simulink model "pendulum_2d_control_simulation"  (R2017a)
settings: Solver=FixedStepAuto  StartTime=0.0  StopTime=15  FixedStep=dt  RelTol=1e-3
values from neighbouring files (symbols this model uses):
  A = [0, 1, 0, 0 ... (first row only)    [formPendel.m]    (also in initialize_controller_pendulum2d.m = double(subs(A_sym)))
  B = [0, 1, 0, -1/L]'    [formPendel.m]    (also in initialize_controller_pendulum2d.m = double(subs(B_sym)))
  C = [1, 0, 0, 0 ... (first row only)    [formPendel.m]    (also in initialize_controller_pendulum2d.m = double(subs(C_sym)))
  D = [0,0]'    [formPendel.m]    (also in initialize_controller_pendulum2d.m = double(subs(D_sym)))
  dt = 1e-3    (= 0.001)    [fJacobian_simulink.m]    (also in formPendel.m; initialize_controller_pendulum2d.m)
  K = lqr(A,B,Q_lqr, R_lqr)    [formPendel.m]    (also in initialize_controller_pendulum2d.m = lqr(A,B,Q_LQR, R_LQR))
  Ke = -KI(1)    [initialize_controller_pendulum2d.m]
  Ko = KI(2:5)    [initialize_controller_pendulum2d.m]
  N = inv(Cm*inv(B*K - A)*B)    [initialize_controller_pendulum2d.m]
  R = diag([0.001^2, 0.01^2])    [formPendel.m]    (also in initialize_controller_pendulum2d.m)
  theta_init = 10*pi/180    (= 0.174532925199)    [formPendel.m]    (also in initialize_controller_pendulum2d.m = 0.349065850399)
  x0 = [0; 0; 0; 0]    [initialize_controller_pendulum2d.m]
  x_init = 0    [formPendel.m]    (also in initialize_controller_pendulum2d.m)
undefined symbols (not defined in the file or in its folder): Continuous, Time
libraries: sharedTrackingLibrary x3, ctrlSharedLib x1
settings Model: Creator=Workstation  LastModifiedBy=Jan

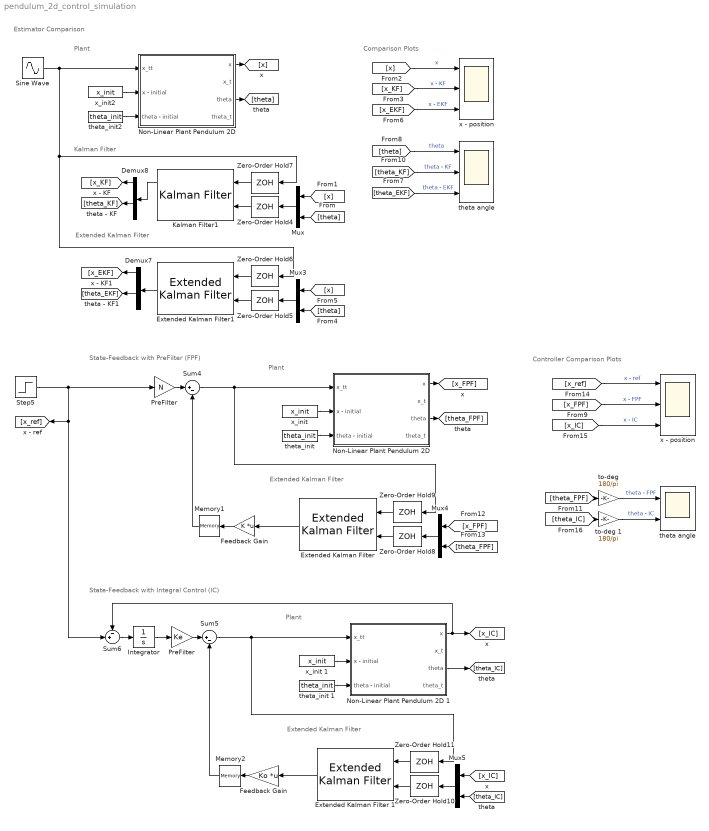
== system pendulum_2d_control_simulation ==
  note: Controller Comparison Plots
  note: Estimator Comparison
  note: State-Feedback with PreFilter (FPF)
  note: Comparison Plots
  note: Extended Kalman Filter
  note: Kalman Filter
  note: Plant
  note: Extended Kalman Filter
  note: Plant
  note: State-Feedback with Integral Control (IC)
  note: Extended Kalman Filter
  note: Plant
  " PreFilter " : Gain  Gain=Ke
  Demux7 : Demux
  Demux8 : Demux
  "Extended Kalman Filter " : sharedTrackingLibrary/Extended Kalman Filter  StateTransitionFcn=f_simulink  HasStateTransitionJacobianFcn=off  HasAdditiveProcessNoise=Additive  ProcessNoise=Q  HasTimeVaryingProcessNoise=off  HasStateTransitionFcnExtraArgument=1  InitialState=x0  InitialStateCovariance=P  MeasurementFcn1=h_simulink  HasMeasurementJacobianFcn1=off  HasMeasurementEnablePort1=off  HasAdditiveMeasurementNoise1=Additive  MeasurementNoise1=R  HasTimeVaryingMeasurementNoise1=off  HasMeasurementFcnExtraArgument1=0  MeasurementFcn2=myMeasurementFcn  HasMeasurementJacobianFcn2=off  HasMeasurementEnablePort2=off  HasAdditiveMeasurementNoise2=Additive  MeasurementNoise2=1  HasTimeVaryingMeasurementNoise2=off  HasMeasurementFcnExtraArgument2=0  MeasurementFcn3=myMeasurementFcn  HasMeasurementJacobianFcn3=off  HasMeasurementEnablePort3=off  HasAdditiveMeasurementNoise3=Additive  MeasurementNoise3=1  HasTimeVaryingMeasurementNoise3=off  HasMeasurementFcnExtraArgument3=0  MeasurementFcn4=myMeasurementFcn  HasMeasurementJacobianFcn4=off  HasMeasurementEnablePort4=off  HasAdditiveMeasurementNoise4=Additive  MeasurementNoise4=1  HasTimeVaryingMeasurementNoise4=off  HasMeasurementFcnExtraArgument4=0  MeasurementFcn5=myMeasurementFcn  HasMeasurementJacobianFcn5=off  HasMeasurementEnablePort5=off  HasAdditiveMeasurementNoise5=Additive  MeasurementNoise5=1  HasTimeVaryingMeasurementNoise5=off  HasMeasurementFcnExtraArgument5=0  EnableMultirate=off  StateTransitionFcnSampleTime=1  MeasurementFcn1SampleTime=1  MeasurementFcn2SampleTime=1  MeasurementFcn3SampleTime=1  MeasurementFcn4SampleTime=1  MeasurementFcn5SampleTime=1  UseCurrentEstimator=on  OutputStateCovariance=off  DataType=double  SampleTime=dt  NumberOfMeasurements=1
  Extended Kalman Filter 1 : sharedTrackingLibrary/Extended Kalman Filter  StateTransitionFcn=f_simulink  HasStateTransitionJacobianFcn=off  HasAdditiveProcessNoise=Additive  ProcessNoise=Q  HasTimeVaryingProcessNoise=off  HasStateTransitionFcnExtraArgument=1  InitialState=x0  InitialStateCovariance=P  MeasurementFcn1=h_simulink  HasMeasurementJacobianFcn1=off  HasMeasurementEnablePort1=off  HasAdditiveMeasurementNoise1=Additive  MeasurementNoise1=R  HasTimeVaryingMeasurementNoise1=off  HasMeasurementFcnExtraArgument1=0  MeasurementFcn2=myMeasurementFcn  HasMeasurementJacobianFcn2=off  HasMeasurementEnablePort2=off  HasAdditiveMeasurementNoise2=Additive  MeasurementNoise2=1  HasTimeVaryingMeasurementNoise2=off  HasMeasurementFcnExtraArgument2=0  MeasurementFcn3=myMeasurementFcn  HasMeasurementJacobianFcn3=off  HasMeasurementEnablePort3=off  HasAdditiveMeasurementNoise3=Additive  MeasurementNoise3=1  HasTimeVaryingMeasurementNoise3=off  HasMeasurementFcnExtraArgument3=0  MeasurementFcn4=myMeasurementFcn  HasMeasurementJacobianFcn4=off  HasMeasurementEnablePort4=off  HasAdditiveMeasurementNoise4=Additive  MeasurementNoise4=1  HasTimeVaryingMeasurementNoise4=off  HasMeasurementFcnExtraArgument4=0  MeasurementFcn5=myMeasurementFcn  HasMeasurementJacobianFcn5=off  HasMeasurementEnablePort5=off  HasAdditiveMeasurementNoise5=Additive  MeasurementNoise5=1  HasTimeVaryingMeasurementNoise5=off  HasMeasurementFcnExtraArgument5=0  EnableMultirate=off  StateTransitionFcnSampleTime=1  MeasurementFcn1SampleTime=1  MeasurementFcn2SampleTime=1  MeasurementFcn3SampleTime=1  MeasurementFcn4SampleTime=1  MeasurementFcn5SampleTime=1  UseCurrentEstimator=on  OutputStateCovariance=off  DataType=double  SampleTime=dt  NumberOfMeasurements=1
  Extended Kalman Filter1 : sharedTrackingLibrary/Extended Kalman Filter  StateTransitionFcn=f_simulink  HasStateTransitionJacobianFcn=off  HasAdditiveProcessNoise=Additive  ProcessNoise=Q  HasTimeVaryingProcessNoise=off  HasStateTransitionFcnExtraArgument=1  InitialState=x0  InitialStateCovariance=P  MeasurementFcn1=h_simulink  HasMeasurementJacobianFcn1=off  HasMeasurementEnablePort1=off  HasAdditiveMeasurementNoise1=Additive  MeasurementNoise1=R  HasTimeVaryingMeasurementNoise1=off  HasMeasurementFcnExtraArgument1=0  MeasurementFcn2=myMeasurementFcn  HasMeasurementJacobianFcn2=off  HasMeasurementEnablePort2=off  HasAdditiveMeasurementNoise2=Additive  MeasurementNoise2=1  HasTimeVaryingMeasurementNoise2=off  HasMeasurementFcnExtraArgument2=0  MeasurementFcn3=myMeasurementFcn  HasMeasurementJacobianFcn3=off  HasMeasurementEnablePort3=off  HasAdditiveMeasurementNoise3=Additive  MeasurementNoise3=1  HasTimeVaryingMeasurementNoise3=off  HasMeasurementFcnExtraArgument3=0  MeasurementFcn4=myMeasurementFcn  HasMeasurementJacobianFcn4=off  HasMeasurementEnablePort4=off  HasAdditiveMeasurementNoise4=Additive  MeasurementNoise4=1  HasTimeVaryingMeasurementNoise4=off  HasMeasurementFcnExtraArgument4=0  MeasurementFcn5=myMeasurementFcn  HasMeasurementJacobianFcn5=off  HasMeasurementEnablePort5=off  HasAdditiveMeasurementNoise5=Additive  MeasurementNoise5=1  HasTimeVaryingMeasurementNoise5=off  HasMeasurementFcnExtraArgument5=0  EnableMultirate=off  StateTransitionFcnSampleTime=1  MeasurementFcn1SampleTime=1  MeasurementFcn2SampleTime=1  MeasurementFcn3SampleTime=1  MeasurementFcn4SampleTime=1  MeasurementFcn5SampleTime=1  UseCurrentEstimator=on  OutputStateCovariance=off  DataType=double  SampleTime=dt  NumberOfMeasurements=1
  Feedback Gain : Gain  Gain=Ko  Multiplication=Matrix(K*u)
  "Feedback Gain " : Gain  Gain=K  Multiplication=Matrix(K*u)
  Integrator : Integrator
  Kalman Filter1 : ctrlSharedLib/Kalman Filter  TimeDomain=Continuous-Time  UseCurrentEstimator=off  ModelSource=Individual A, B, C, D matrices  ModelSourceVariable=ss(0.95,1,1,0,1)  A=A  B=B  C=C  D=D  NumberOfStates=1  NumberOfInputs=1  NumberOfOutputs=1  InitialEstimateSource=Dialog  X0=x0  P0=10  UseK=off  UseGH=off  NumberOfProcessNoiseInputs=1  G=1  TimeInvariantG=on  H=0  TimeInvariantH=on  Q=Q  TimeInvariantQ=on  R=R  TimeInvariantR=on  N=0  TimeInvariantN=on  AddInputPort=on  AddEnablePort=off  ExternalReset=none  OutputEstimatedY=on  OutputP=off  Ts=dt
  Memory1 : Memory
  Memory2 : Memory
  Mux{,3..5} (4 alike) : Mux  Inputs=2
  Non-Linear Plant Pendulum 2D : Subsystem
  "Non-Linear Plant Pendulum 2D " : Subsystem
  Non-Linear Plant Pendulum 2D 1 : Subsystem
  PreFilter : Gain  Gain=N
  Sine Wave : Sin  SampleTime=0
  Step5 : Step  Time=0  SampleTime=0
  Sum4 : Sum  Inputs=|+-
  Sum5 : Sum  Inputs=|+-
  Sum6 : Sum  Inputs=-+|
  Zero-Order Hold{5..6,8..11} (6 alike) : ZeroOrderHold  SampleTime=dt
  Zero-Order Hold4 : ZeroOrderHold  SampleTime=-1
  Zero-Order Hold7 : ZeroOrderHold  SampleTime=-1
  theta angle : Scope  NumInputPorts=3
  "theta angle " : Scope  NumInputPorts=2
  "theta_init " : Constant  Value=theta_init
  theta_init 1 : Constant  Value=theta_init
  theta_init2 : Constant  Value=theta_init
  "to-deg " : Gain  Gain=180/pi
  to-deg 1 : Gain  Gain=180/pi
  x - position : Scope  NumInputPorts=3
  "x - position " : Scope  NumInputPorts=3
  "x_init " : Constant  Value=x_init
  x_init 1 : Constant  Value=x_init
  x_init2 : Constant  Value=x_init
  wires:
  x_init2/1 -> Non-Linear Plant Pendulum 2D/2(x - initial)
  theta_init2/1 -> Non-Linear Plant Pendulum 2D/3(theta - initial)
  Non-Linear Plant Pendulum 2D/3(theta) -> [theta]
  Non-Linear Plant Pendulum 2D/1(x) -> [x]
  Mux/1 -> Zero-Order Hold4/1
  Zero-Order Hold4/1 -> Kalman Filter1/2
  [theta] -> Mux/2
  [x] -> Mux/1
  [x] -> x - position/1  "x"
  [x_KF] -> x - position/2  "x - KF"
  Zero-Order Hold5/1 -> Extended Kalman Filter1/2
  [x] -> Mux3/1
  [theta] -> Mux3/2
  Mux3/1 -> Zero-Order Hold5/1
  Extended Kalman Filter1/1 -> Demux7/1
  Demux7/1 -> [x_EKF]
  [x_EKF] -> x - position/3  "x - EKF"
  Demux7/3 -> [theta_EKF]
  Kalman Filter1/1 -> Demux8/1
  Demux8/1 -> [x_KF]
  Demux8/3 -> [theta_KF]
  Zero-Order Hold7/1 -> Kalman Filter1/1
  Zero-Order Hold6/1 -> Extended Kalman Filter1/1
  Sine Wave/1 -> Non-Linear Plant Pendulum 2D/1(x_tt), Zero-Order Hold6/1, Zero-Order Hold7/1
  [theta_KF] -> theta angle/2  "theta - KF"
  [theta_EKF] -> theta angle/3  "theta - EKF"
  [theta] -> theta angle/1  "theta"
  Zero-Order Hold9/1 -> "Extended Kalman Filter "/1
  "Extended Kalman Filter "/1 -> "Feedback Gain "/1
  Mux4/1 -> Zero-Order Hold8/1
  [theta_FPF] -> Mux4/2
  [x_FPF] -> Mux4/1
  Zero-Order Hold8/1 -> "Extended Kalman Filter "/2
  "Non-Linear Plant Pendulum 2D "/1(x) -> [x_FPF]
  "Non-Linear Plant Pendulum 2D "/3(theta) -> [theta_FPF]
  "theta_init "/1 -> "Non-Linear Plant Pendulum 2D "/3(theta - initial)
  "x_init "/1 -> "Non-Linear Plant Pendulum 2D "/2(x - initial)
  Sum4/1 -> Zero-Order Hold9/1, "Non-Linear Plant Pendulum 2D "/1(x_tt)
  "Feedback Gain "/1 -> Memory1/1
  Memory1/1 -> Sum4/2
  PreFilter/1 -> Sum4/1
  [theta_FPF] -> "to-deg "/1
  [x_FPF] -> "x - position "/2  "x - FPF"
  [x_ref] -> "x - position "/1  "x - ref"
  "to-deg "/1 -> "theta angle "/1  "theta - FPF"
  Integrator/1 -> " PreFilter "/1
  " PreFilter "/1 -> Sum5/1
  Memory2/1 -> Sum5/2
  Feedback Gain/1 -> Memory2/1
  Sum5/1 -> Non-Linear Plant Pendulum 2D 1/1(x_tt), Zero-Order Hold11/1
  x_init 1/1 -> Non-Linear Plant Pendulum 2D 1/2(x - initial)
  theta_init 1/1 -> Non-Linear Plant Pendulum 2D 1/3(theta - initial)
  Non-Linear Plant Pendulum 2D 1/3(theta) -> [theta_IC]
  Zero-Order Hold10/1 -> Extended Kalman Filter 1/2
  [x_IC] -> Mux5/1
  [theta_IC] -> Mux5/2
  Mux5/1 -> Zero-Order Hold10/1
  Extended Kalman Filter 1/1 -> Feedback Gain/1
  Zero-Order Hold11/1 -> Extended Kalman Filter 1/1
  Sum6/1 -> Integrator/1
  Non-Linear Plant Pendulum 2D 1/1(x) -> [x_IC], Sum6/1
  [x_IC] -> "x - position "/3  "x - IC"
  [theta_IC] -> to-deg 1/1
  to-deg 1/1 -> "theta angle "/2  "theta - IC"
  Step5/1 -> PreFilter/1, [x_ref], Sum6/2

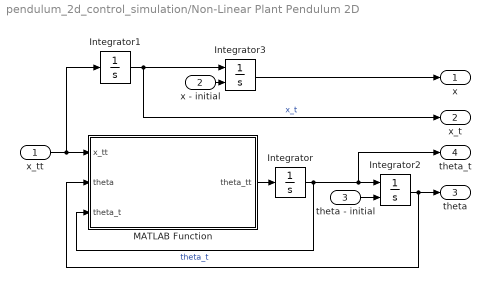
== system pendulum_2d_control_simulation/Non-Linear Plant Pendulum 2D ==
  x_tt : Inport
  x - initial : Inport  Port=2
  theta - initial : Inport  Port=3
  Integrator : Integrator
  Integrator1 : Integrator
  Integrator2 : Integrator  InitialConditionSource=external
  Integrator3 : Integrator  InitialConditionSource=external
  MATLAB Function : MATLAB Function  TreatAsAtomicUnit=on
  x : Outport
  x_t : Outport  Port=2
  theta : Outport  Port=3
  theta_t : Outport  Port=4
  wires:
  Integrator/1 -> MATLAB Function/3(theta_t), theta_t/1, Integrator2/1  "theta_t"
  x_tt/1 -> MATLAB Function/1(x_tt), Integrator1/1
  x - initial/1 -> Integrator3/2
  Integrator1/1 -> Integrator3/1, x_t/1  "x_t"
  MATLAB Function/1(theta_tt) -> Integrator/1
  theta - initial/1 -> Integrator2/2
  Integrator2/1 -> MATLAB Function/2(theta), theta/1
  Integrator3/1 -> x/1

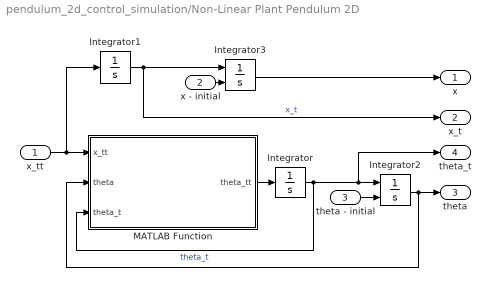
== system pendulum_2d_control_simulation/Non-Linear Plant Pendulum 2D  ==
  x_tt : Inport
  x - initial : Inport  Port=2
  theta - initial : Inport  Port=3
  Integrator : Integrator
  Integrator1 : Integrator
  Integrator2 : Integrator  InitialConditionSource=external
  Integrator3 : Integrator  InitialConditionSource=external
  MATLAB Function : MATLAB Function  TreatAsAtomicUnit=on
  x : Outport
  x_t : Outport  Port=2
  theta : Outport  Port=3
  theta_t : Outport  Port=4
  wires:
  Integrator3/1 -> x/1
  Integrator2/1 -> theta/1, MATLAB Function/2(theta)
  theta - initial/1 -> Integrator2/2
  MATLAB Function/1(theta_tt) -> Integrator/1
  Integrator1/1 -> x_t/1, Integrator3/1  "x_t"
  x - initial/1 -> Integrator3/2
  x_tt/1 -> Integrator1/1, MATLAB Function/1(x_tt)
  Integrator/1 -> Integrator2/1, theta_t/1, MATLAB Function/3(theta_t)  "theta_t"

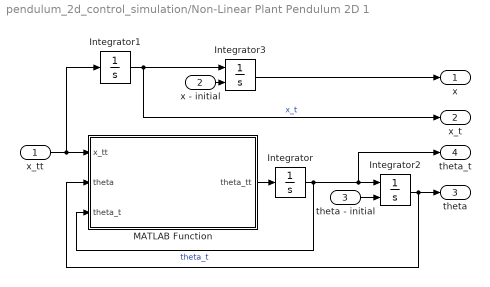
== system pendulum_2d_control_simulation/Non-Linear Plant Pendulum 2D 1 ==
  x_tt : Inport
  x - initial : Inport  Port=2
  theta - initial : Inport  Port=3
  Integrator : Integrator
  Integrator1 : Integrator
  Integrator2 : Integrator  InitialConditionSource=external
  Integrator3 : Integrator  InitialConditionSource=external
  MATLAB Function : MATLAB Function  TreatAsAtomicUnit=on
  x : Outport
  x_t : Outport  Port=2
  theta : Outport  Port=3
  theta_t : Outport  Port=4
  wires:
  Integrator/1 -> MATLAB Function/3(theta_t), theta_t/1, Integrator2/1  "theta_t"
  x_tt/1 -> MATLAB Function/1(x_tt), Integrator1/1
  x - initial/1 -> Integrator3/2
  Integrator1/1 -> Integrator3/1, x_t/1  "x_t"
  MATLAB Function/1(theta_tt) -> Integrator/1
  theta - initial/1 -> Integrator2/2
  Integrator2/1 -> MATLAB Function/2(theta), theta/1
  Integrator3/1 -> x/1

== matlab function pendulum_2d_control_simulation/Non-Linear Plant Pendulum 2D/MATLAB Function ==
  data: x_tt input; theta input; theta_tt output; theta_t input
function theta_tt = pendulum_dynamics(x_tt, theta, theta_t)
    
    % Constants
    g = 9.81;   % Gravity
    L = 2.0;    % Wire length
    
    % Pendulum ODE
    theta_tt = (-g*sin(theta) - cos(theta)*x_tt)/(L);

== matlab function pendulum_2d_control_simulation/Non-Linear Plant Pendulum 2D /MATLAB Function ==
  data: x_tt input; theta input; theta_tt output; theta_t input
function theta_tt = pendulum_dynamics(x_tt, theta, theta_t)
    
    % Constants
    g = 9.81;   % Gravity
    L = 2.0;    % Wire length
    
    % Pendulum ODE
    theta_tt = (-g*sin(theta) - cos(theta)*x_tt)/(L);

== matlab function pendulum_2d_control_simulation/Non-Linear Plant Pendulum 2D 1/MATLAB Function ==
  data: x_tt input; theta input; theta_tt output; theta_t input
function theta_tt = pendulum_dynamics(x_tt, theta, theta_t)
    
    % Constants
    g = 9.81;   % Gravity
    L = 2.0;    % Wire length
    
    % Pendulum ODE
    theta_tt = (-g*sin(theta) - cos(theta)*x_tt)/(L);
